simulink model "Diff_TrqRat"  (R2016b)
settings: configuration reference "CodeGenConfigSet" (kept outside this file)
values from neighbouring files (symbols this model uses):
  Diff_rTrqDfftl_C = Calibration.Parameter    [init_Diff_TrqRat.m]    (also in init_Diff_TrqRat_SIL.m = Simulink.Parameter)
  DiffIO_rTrqDfftl_C = Calibration.Parameter    [init_Diff_TrqRat.m]    (also in init_Diff_TrqRat_SIL.m = Simulink.Parameter)
settings Model: Creator=Administrator  LastModifiedBy=Wollf
settings ConfigSetRef: SourceLocation=Base Workspace

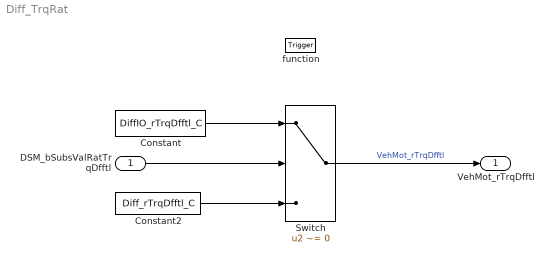
== system Diff_TrqRat ==
  DSM_bSubsValRatTrqDfftl : Inport  Description=Status of FId_SubsValRatTrqDfftl  OutMin=0  OutMax=1  OutDataTypeStr=boolean
  function : TriggerPort  TriggerType=function-call  VariantControl=Variant
  Constant : Constant  Value=DiffIO_rTrqDfftl_C
  Constant2 : Constant  Value=Diff_rTrqDfftl_C
  Switch : Switch  Criteria=u2 ~= 0  InputSameDT=on
  VehMot_rTrqDfftl : Outport  Description=Torque ratio of differential  OutMin=-300  OutMax=300  OutDataTypeStr=TransRatio
  wires:
  Constant2/1 -> Switch/3
  DSM_bSubsValRatTrqDfftl/1 -> Switch/2
  Switch/1 -> VehMot_rTrqDfftl/1  "VehMot_rTrqDfftl"
  Constant/1 -> Switch/1
